simulink model "Case1_Sim"  (R2020b)
settings: Solver=FixedStepAuto  StartTime=0.0  StopTime=0.8  FixedStep=Ts  RelTol=1e-3
values from neighbouring files (symbols this model uses):
  m = 5/100    (= 0.05)    [Case1_SimPara.m]
  Sbase = 1    [Case1_SimPara.m]
  Ts = 1/Fs    (= 0.0001)    [Case1_SimPara.m]
  Vbase = 1    [Case1_SimPara.m]
  w_droop = 10*2*pi    (= 62.8318530718)    [Case1_SimPara.m]
  w_pll = 10*2*pi    (= 62.8318530718)    [Case1_SimPara.m]
  w_tau = 1e3*2*pi    (= 6283.18530718)    [Case1_SimPara.m]
  Wbase = 2*pi*50    (= 314.159265359)    [Case1_SimPara.m]
undefined symbols (not defined in the file or in its folder): DiscIntNeverNeededParam
libraries: SimplexPS x22, powerlib x1
(part 1 of 2)
settings Model: Creator=admin_user  LastModifiedBy=admin_user
settings DataIOCC: ReturnWorkspaceOutputs=off

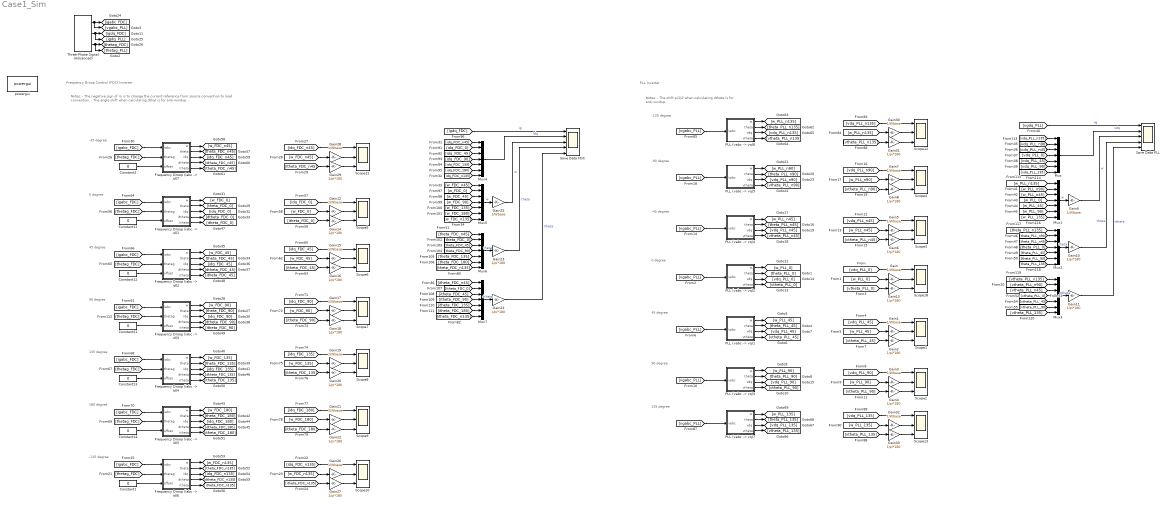
== system Case1_Sim ==
  note: Notes:
      | - The shift pi/2/2 when calculating dtheta is for anti-windup.
  note: Notes:
      | - The negative sign of m is to change the current reference from source convention to load convention.
      | - The angle shift when calculating dthat is for anti-windup.
  note: Frequency Droop Control (FDC) Inverter
  note: 0 degree
  note: PLL Inverter
  note: 90 degree
  note: 0 degree
  note: 45 degree
  note: 135 degree
  note: 180 degree
  note: 45 degree
  note: 90 degree
  note: -45 degree
  note: -90 degree
  note: -135 degree
  note: -45 degree
  note: -135 degree
  note: 135 degree
  Constant{1..2,11..14,21} (7 alike) : Constant  Value=0
  "Frequency Droop (iabc -> id)1" : Subsystem  AncestorBlock=|  mask{Ts=Ts, Sbase=Sbase, Vbase=Vbase, Wbase=Wbase, m=-m, w_tau=w_droop, theta0=0, i0=0, w0=1}
      | SimplexPS/Frequency Droop
      | (iabc -> id)
      mask prompts: Ts "Ts (s), samping period"; Sbase "Sbase (VA), base power"; Vbase "Vbase (V), base voltage"; Wbase "Wbase (rad/s), base angular frequency"; m "m (pu), droop gain"; w_tau "w_tau (rad/s), low-pass filter bandwidth"; theta0 "theta0 (rad), initial angle"; i0 "i0 (pu), current setting point"; w0 "w0 (pu), frequency setting point"
  "Frequency Droop (iabc -> id)2" : Subsystem  AncestorBlock=|  mask{Ts=Ts, Sbase=Sbase, Vbase=Vbase, Wbase=Wbase, m=-m, w_tau=w_droop, theta0=pi/2/2, i0=0, w0=1}
      | SimplexPS/Frequency Droop
      | (iabc -> id)
      mask prompts: Ts "Ts (s), samping period"; Sbase "Sbase (VA), base power"; Vbase "Vbase (V), base voltage"; Wbase "Wbase (rad/s), base angular frequency"; m "m (pu), droop gain"; w_tau "w_tau (rad/s), low-pass filter bandwidth"; theta0 "theta0 (rad), initial angle"; i0 "i0 (pu), current setting point"; w0 "w0 (pu), frequency setting point"
  "Frequency Droop (iabc -> id)3" : Subsystem  AncestorBlock=|  mask{Ts=Ts, Sbase=Sbase, Vbase=Vbase, Wbase=Wbase, m=-m, w_tau=w_droop, theta0=pi/2, i0=0, w0=1}
      | SimplexPS/Frequency Droop
      | (iabc -> id)
      mask prompts: Ts "Ts (s), samping period"; Sbase "Sbase (VA), base power"; Vbase "Vbase (V), base voltage"; Wbase "Wbase (rad/s), base angular frequency"; m "m (pu), droop gain"; w_tau "w_tau (rad/s), low-pass filter bandwidth"; theta0 "theta0 (rad), initial angle"; i0 "i0 (pu), current setting point"; w0 "w0 (pu), frequency setting point"
  "Frequency Droop (iabc -> id)4" : Subsystem  AncestorBlock=|  mask{Ts=Ts, Sbase=Sbase, Vbase=Vbase, Wbase=Wbase, m=-m, w_tau=w_droop, theta0=pi/2/2*3, i0=0, w0=1}
      | SimplexPS/Frequency Droop
      | (iabc -> id)
      mask prompts: Ts "Ts (s), samping period"; Sbase "Sbase (VA), base power"; Vbase "Vbase (V), base voltage"; Wbase "Wbase (rad/s), base angular frequency"; m "m (pu), droop gain"; w_tau "w_tau (rad/s), low-pass filter bandwidth"; theta0 "theta0 (rad), initial angle"; i0 "i0 (pu), current setting point"; w0 "w0 (pu), frequency setting point"
  "Frequency Droop (iabc -> id)5" : Subsystem  AncestorBlock=|  mask{Ts=Ts, Sbase=Sbase, Vbase=Vbase, Wbase=Wbase, m=-m, w_tau=w_droop, theta0=pi, i0=0, w0=1}
      | SimplexPS/Frequency Droop
      | (iabc -> id)
      mask prompts: Ts "Ts (s), samping period"; Sbase "Sbase (VA), base power"; Vbase "Vbase (V), base voltage"; Wbase "Wbase (rad/s), base angular frequency"; m "m (pu), droop gain"; w_tau "w_tau (rad/s), low-pass filter bandwidth"; theta0 "theta0 (rad), initial angle"; i0 "i0 (pu), current setting point"; w0 "w0 (pu), frequency setting point"
  "Frequency Droop (iabc -> id)6" : Subsystem  AncestorBlock=|  mask{Ts=Ts, Sbase=Sbase, Vbase=Vbase, Wbase=Wbase, m=-m, w_tau=w_droop, theta0=-pi/2/2*3, i0=0, w0=1}
      | SimplexPS/Frequency Droop
      | (iabc -> id)
      mask prompts: Ts "Ts (s), samping period"; Sbase "Sbase (VA), base power"; Vbase "Vbase (V), base voltage"; Wbase "Wbase (rad/s), base angular frequency"; m "m (pu), droop gain"; w_tau "w_tau (rad/s), low-pass filter bandwidth"; theta0 "theta0 (rad), initial angle"; i0 "i0 (pu), current setting point"; w0 "w0 (pu), frequency setting point"
  "Frequency Droop (iabc -> id)7" : Subsystem  AncestorBlock=|  mask{Ts=Ts, Sbase=Sbase, Vbase=Vbase, Wbase=Wbase, m=-m, w_tau=w_droop, theta0=-pi/2/2, i0=0, w0=1}
      | SimplexPS/Frequency Droop
      | (iabc -> id)
      mask prompts: Ts "Ts (s), samping period"; Sbase "Sbase (VA), base power"; Vbase "Vbase (V), base voltage"; Wbase "Wbase (rad/s), base angular frequency"; m "m (pu), droop gain"; w_tau "w_tau (rad/s), low-pass filter bandwidth"; theta0 "theta0 (rad), initial angle"; i0 "i0 (pu), current setting point"; w0 "w0 (pu), frequency setting point"
  Gain{,1,3,5,7,9,12,15,17,19,21,25..26,28,30,32} (16 alike) : Gain  Gain=1/Wbase
  Gain{2,4,6,8,10..11,13..14,16,18,20,22..24,27,29,31,33} (18 alike) : Gain  Gain=1/pi*180
  Mux : Mux  Inputs=[2,2,2,2,2,2,2]
  Mux{1..3,5..7} (6 alike) : Mux  Inputs=7
  Mux4 : Mux  Inputs=[2,2,2,2,2,2,2]
  "PLL (vabc -> vq)1" : Subsystem  AncestorBlock=|  mask{Ts=Ts, Vbase=Vbase, Wbase=Wbase, w_pll=w_pll, w_tau=w_tau, theta0=pi/2/2}
      | SimplexPS/PLL
      | (vabc -> vq)
      mask prompts: Ts "Ts (s), sampling period"; Vbase "Vbase (V), base voltage"; Wbase "Wbase (rad/s), base angular frequency"; w_pll "w_pll (rad/s), PLL bandwidth"; w_tau "w_tau (rad/s), low-pass filter bandwidth"; theta0 "theta0 (rad), initial angle"
  "PLL (vabc -> vq)2" : Subsystem  AncestorBlock=|  mask{Ts=Ts, Vbase=Vbase, Wbase=Wbase, w_pll=w_pll, w_tau=w_tau, theta0=0}
      | SimplexPS/PLL
      | (vabc -> vq)
      mask prompts: Ts "Ts (s), sampling period"; Vbase "Vbase (V), base voltage"; Wbase "Wbase (rad/s), base angular frequency"; w_pll "w_pll (rad/s), PLL bandwidth"; w_tau "w_tau (rad/s), low-pass filter bandwidth"; theta0 "theta0 (rad), initial angle"
  "PLL (vabc -> vq)3" : Subsystem  AncestorBlock=|  mask{Ts=Ts, Vbase=Vbase, Wbase=Wbase, w_pll=w_pll, w_tau=w_tau, theta0=pi/2}
      | SimplexPS/PLL
      | (vabc -> vq)
      mask prompts: Ts "Ts (s), sampling period"; Vbase "Vbase (V), base voltage"; Wbase "Wbase (rad/s), base angular frequency"; w_pll "w_pll (rad/s), PLL bandwidth"; w_tau "w_tau (rad/s), low-pass filter bandwidth"; theta0 "theta0 (rad), initial angle"
  "PLL (vabc -> vq)4" : Subsystem  AncestorBlock=|  mask{Ts=Ts, Vbase=Vbase, Wbase=Wbase, w_pll=w_pll, w_tau=w_tau, theta0=-pi/2/2}
      | SimplexPS/PLL
      | (vabc -> vq)
      mask prompts: Ts "Ts (s), sampling period"; Vbase "Vbase (V), base voltage"; Wbase "Wbase (rad/s), base angular frequency"; w_pll "w_pll (rad/s), PLL bandwidth"; w_tau "w_tau (rad/s), low-pass filter bandwidth"; theta0 "theta0 (rad), initial angle"
  "PLL (vabc -> vq)5" : Subsystem  AncestorBlock=|  mask{Ts=Ts, Vbase=Vbase, Wbase=Wbase, w_pll=w_pll, w_tau=w_tau, theta0=-pi/2}
      | SimplexPS/PLL
      | (vabc -> vq)
      mask prompts: Ts "Ts (s), sampling period"; Vbase "Vbase (V), base voltage"; Wbase "Wbase (rad/s), base angular frequency"; w_pll "w_pll (rad/s), PLL bandwidth"; w_tau "w_tau (rad/s), low-pass filter bandwidth"; theta0 "theta0 (rad), initial angle"
  "PLL (vabc -> vq)6" : Subsystem  AncestorBlock=|  mask{Ts=Ts, Vbase=Vbase, Wbase=Wbase, w_pll=w_pll, w_tau=w_tau, theta0=-pi/2/2*3}
      | SimplexPS/PLL
      | (vabc -> vq)
      mask prompts: Ts "Ts (s), sampling period"; Vbase "Vbase (V), base voltage"; Wbase "Wbase (rad/s), base angular frequency"; w_pll "w_pll (rad/s), PLL bandwidth"; w_tau "w_tau (rad/s), low-pass filter bandwidth"; theta0 "theta0 (rad), initial angle"
  "PLL (vabc -> vq)7" : Subsystem  AncestorBlock=|  mask{Ts=Ts, Vbase=Vbase, Wbase=Wbase, w_pll=w_pll, w_tau=w_tau, theta0=pi/2/2*3}
      | SimplexPS/PLL
      | (vabc -> vq)
      mask prompts: Ts "Ts (s), sampling period"; Vbase "Vbase (V), base voltage"; Wbase "Wbase (rad/s), base angular frequency"; w_pll "w_pll (rad/s), PLL bandwidth"; w_tau "w_tau (rad/s), low-pass filter bandwidth"; theta0 "theta0 (rad), initial angle"
  Save Data FDC : Scope  NumInputPorts=5
  Save Data PLL : Scope  NumInputPorts=5
  Scope{1..13,18} (14 alike) : Scope  NumInputPorts=3
  Three-Phase Signal (Advanced) : SimplexPS/Three-Phase Signal (Advanced)  Ts=Ts  ud=1  uq=0  w=Wbase  theta0=0  enable_freq_step=1  ratio_freq_step=0.96  time_freq_step=0.4
      settings: SourceProductName=Simplex Power Systems
  powergui : powerlib/powergui  Priority=1  SimulationMode=Discrete  SampleTime=Ts  frequency=60  Iterations=50  frequencyindice=0  Pbase=100e6  ErrMax=1e-4  UnitsV=kV  UnitsW=MW  buscounter=0  FunctionMessages=off  echomessages=off  EnableUseOfTLC=off  CurrentSourceSwitches=off  DisableSnubberDevices=off  DisableRonSwitches=off  DisableVfSwitches=off  DisplayEquations=off  AutomaticDiscreteSolvers=off  SolverType=Tustin/Backward Euler (TBE)  Interpol=off  ExternalGateDelay=off  methode=off  Ts=100  x0status=blocks  SPID=on  SwTol=0  HookPort=off  NonlinearTolerance=1e-4  nMaxIteration=100  ContinueOnMaxIteration=off  RestoreLinks=warning  ResistiveCurrentMeasurement=off  Frange=[0:2:500]  Ylog=off  Xlog=on  ShowGrid=off  save=off  variable=ZData  structure=0  ZoomFFT=off  StartTime=0.0  cycles=1  DisplayStyle=1  fundamental=60  FreqAxis=off  MaxFrequency=1000  frequencyindicesteady=1  RmsSteady=1  display=off
  wires:
  Three-Phase Signal (Advanced)/2 -> [igdq_PLL], [igdq_FDC]
  "PLL (vabc -> vq)2"/1(w) -> [w_PLL_0]
  "PLL (vabc -> vq)2"/3(vdq) -> [vdq_PLL_0]
  [vdq_PLL_0] -> Scope18/1
  "PLL (vabc -> vq)2"/2(theta) -> [theta_PLL_0]
  Three-Phase Signal (Advanced)/3 -> [thetag_PLL], [thetag_FDC]
  [w_PLL_0] -> Gain/1
  Three-Phase Signal (Advanced)/1 -> [vgabc_PLL], [igabc_FDC]
  [vgabc_PLL] -> "PLL (vabc -> vq)2"/1(vabc)
  [vgdq_PLL] -> Save Data PLL/1  "vg"
  Mux/1 -> Save Data PLL/2  "vdq"
  Mux1/1 -> Gain9/1  "w"
  Gain9/1 -> Save Data PLL/3  "w"
  Mux2/1 -> Gain10/1  "theta"
  Gain10/1 -> Save Data PLL/4  "theta"
  Mux3/1 -> Gain11/1  "dtheta"
  Gain11/1 -> Save Data PLL/5  "vtheta"
  "Frequency Droop (iabc -> id)3"/2(theta) -> [theta_FDC_90]
  [igabc_FDC] -> "Frequency Droop (iabc -> id)3"/1(iabc)
  "Frequency Droop (iabc -> id)3"/3(idq) -> [idq_FDC_90]
  [w_FDC_0] -> Gain12/1
  [idq_FDC_0] -> Scope5/1
  "Frequency Droop (iabc -> id)3"/1(w) -> [w_FDC_90]
  [vtheta_PLL_0] -> Gain13/1
  [itheta_FDC_0] -> Gain14/1
  Mux4/1 -> Save Data FDC/2  "idq"
  [igdq_FDC] -> Save Data FDC/1  "ig"
  Gain24/1 -> Save Data FDC/5  "itheta"
  Mux5/1 -> Gain25/1  "w"
  Gain23/1 -> Save Data FDC/4  "theta"
  Mux7/1 -> Gain24/1  "dtheta"
  Gain25/1 -> Save Data FDC/3  "w"
  Mux6/1 -> Gain23/1  "theta"
  [thetag_FDC] -> "Frequency Droop (iabc -> id)3"/2(thetag)
  Constant21/1 -> "Frequency Droop (iabc -> id)3"/3(offset)
  "Frequency Droop (iabc -> id)3"/4(dtheta) -> [dtheta_FDC_90]
  Gain12/1 -> Scope5/2
  Gain14/1 -> Scope5/3
  Gain16/1 -> Scope6/3
  Gain15/1 -> Scope6/2
  [w_FDC_45] -> Gain15/1
  [idq_FDC_45] -> Scope6/1
  [itheta_FDC_45] -> Gain16/1
  "Frequency Droop (iabc -> id)1"/3(idq) -> [idq_FDC_0]
  "Frequency Droop (iabc -> id)1"/2(theta) -> [theta_FDC_0]
  "Frequency Droop (iabc -> id)1"/1(w) -> [w_FDC_0]
  [thetag_FDC] -> "Frequency Droop (iabc -> id)1"/2(thetag)
  "Frequency Droop (iabc -> id)1"/4(dtheta) -> [dtheta_FDC_0]
  [igabc_FDC] -> "Frequency Droop (iabc -> id)1"/1(iabc)
  Constant11/1 -> "Frequency Droop (iabc -> id)1"/3(offset)
  Constant12/1 -> "Frequency Droop (iabc -> id)2"/3(offset)
  [igabc_FDC] -> "Frequency Droop (iabc -> id)2"/1(iabc)
  "Frequency Droop (iabc -> id)2"/1(w) -> [w_FDC_45]
  "Frequency Droop (iabc -> id)2"/2(theta) -> [theta_FDC_45]
  "Frequency Droop (iabc -> id)2"/3(idq) -> [idq_FDC_45]
  [thetag_FDC] -> "Frequency Droop (iabc -> id)2"/2(thetag)
  "Frequency Droop (iabc -> id)2"/4(dtheta) -> [dtheta_FDC_45]
  Constant13/1 -> "Frequency Droop (iabc -> id)4"/3(offset)
  "Frequency Droop (iabc -> id)4"/4(dtheta) -> [dtheta_FDC_135]
  [thetag_FDC] -> "Frequency Droop (iabc -> id)4"/2(thetag)
  [igabc_FDC] -> "Frequency Droop (iabc -> id)4"/1(iabc)
  "Frequency Droop (iabc -> id)4"/2(theta) -> [theta_FDC_135]
  "Frequency Droop (iabc -> id)4"/1(w) -> [w_FDC_135]
  "Frequency Droop (iabc -> id)4"/3(idq) -> [idq_FDC_135]
  [thetag_FDC] -> "Frequency Droop (iabc -> id)5"/2(thetag)
  "Frequency Droop (iabc -> id)5"/1(w) -> [w_FDC_180]
  [igabc_FDC] -> "Frequency Droop (iabc -> id)5"/1(iabc)
  "Frequency Droop (iabc -> id)5"/2(theta) -> [theta_FDC_180]
  "Frequency Droop (iabc -> id)5"/4(dtheta) -> [dtheta_FDC_180]
  "Frequency Droop (iabc -> id)5"/3(idq) -> [idq_FDC_180]
  Constant14/1 -> "Frequency Droop (iabc -> id)5"/3(offset)
  Gain18/1 -> Scope7/3
  [idq_FDC_90] -> Scope7/1
  [itheta_FDC_90] -> Gain18/1
  Gain17/1 -> Scope7/2
  [w_FDC_90] -> Gain17/1
  [itheta_FDC_135] -> Gain20/1
  Gain19/1 -> Scope8/2
  Gain20/1 -> Scope8/3
  [w_FDC_135] -> Gain19/1
  [idq_FDC_135] -> Scope8/1
  [idq_FDC_180] -> Scope9/1
  [itheta_FDC_180] -> Gain22/1
  Gain22/1 -> Scope9/3
  Gain21/1 -> Scope9/2
  [w_FDC_180] -> Gain21/1
  "Frequency Droop (iabc -> id)1"/5(itheta) -> [itheta_FDC_0]
  "Frequency Droop (iabc -> id)2"/5(itheta) -> [itheta_FDC_45]
  "Frequency Droop (iabc -> id)3"/5(itheta) -> [itheta_FDC_90]
  "Frequency Droop (iabc -> id)4"/5(itheta) -> [itheta_FDC_135]
  "Frequency Droop (iabc -> id)5"/5(itheta) -> [itheta_FDC_180]
  "PLL (vabc -> vq)2"/4(vtheta) -> [vtheta_PLL_0]
  Gain/1 -> Scope18/2
  Gain13/1 -> Scope18/3
  Gain1/1 -> Scope1/2
  Gain2/1 -> Scope1/3
  [w_PLL_45] -> Gain1/1
  "PLL (vabc -> vq)1"/1(w) -> [w_PLL_45]
  "PLL (vabc -> vq)1"/2(theta) -> [theta_PLL_45]
  "PLL (vabc -> vq)1"/3(vdq) -> [vdq_PLL_45]
  [vgabc_PLL] -> "PLL (vabc -> vq)1"/1(vabc)
  [vdq_PLL_45] -> Scope1/1
  "PLL (vabc -> vq)1"/4(vtheta) -> [vtheta_PLL_45]
  [vtheta_PLL_45] -> Gain2/1
  Gain3/1 -> Scope2/2
  Gain4/1 -> Scope2/3
  [w_PLL_90] -> Gain3/1
  "PLL (vabc -> vq)3"/1(w) -> [w_PLL_90]
  "PLL (vabc -> vq)3"/2(theta) -> [theta_PLL_90]
  "PLL (vabc -> vq)3"/3(vdq) -> [vdq_PLL_90]
  [vgabc_PLL] -> "PLL (vabc -> vq)3"/1(vabc)
  [vdq_PLL_90] -> Scope2/1
  "PLL (vabc -> vq)3"/4(vtheta) -> [vtheta_PLL_90]
  [vtheta_PLL_90] -> Gain4/1
  Gain5/1 -> Scope3/2
  Gain6/1 -> Scope3/3
  [w_PLL_n45] -> Gain5/1
  "PLL (vabc -> vq)4"/1(w) -> [w_PLL_n45]
  "PLL (vabc -> vq)4"/2(theta) -> [theta_PLL_n45]
  "PLL (vabc -> vq)4"/3(vdq) -> [vdq_PLL_n45]
  [vgabc_PLL] -> "PLL (vabc -> vq)4"/1(vabc)
  [vdq_PLL_n45] -> Scope3/1
  "PLL (vabc -> vq)4"/4(vtheta) -> [vtheta_PLL_n45]
  [vtheta_PLL_n45] -> Gain6/1
  [w_PLL_n90] -> Gain7/1
  Gain8/1 -> Scope4/3
  "PLL (vabc -> vq)5"/4(vtheta) -> [vtheta_PLL_n90]
  "PLL (vabc -> vq)5"/2(theta) -> [theta_PLL_n90]
  [vdq_PLL_n90] -> Scope4/1
  [vgabc_PLL] -> "PLL (vabc -> vq)5"/1(vabc)
  "PLL (vabc -> vq)5"/1(w) -> [w_PLL_n90]
  [vtheta_PLL_n90] -> Gain8/1
  "PLL (vabc -> vq)5"/3(vdq) -> [vdq_PLL_n90]
  Gain7/1 -> Scope4/2
  "Frequency Droop (iabc -> id)6"/5(itheta) -> [itheta_FDC_n135]
  Gain26/1 -> Scope10/2
  [idq_FDC_n135] -> Scope10/1
  [itheta_FDC_n135] -> Gain27/1
  Constant1/1 -> "Frequency Droop (iabc -> id)6"/3(offset)
  [igabc_FDC] -> "Frequency Droop (iabc -> id)6"/1(iabc)
  "Frequency Droop (iabc -> id)6"/1(w) -> [w_FDC_n135]
  Gain27/1 -> Scope10/3
  "Frequency Droop (iabc -> id)6"/2(theta) -> [theta_FDC_n135]
  [thetag_FDC] -> "Frequency Droop (iabc -> id)6"/2(thetag)
  "Frequency Droop (iabc -> id)6"/4(dtheta) -> [dtheta_FDC_n135]
  [w_FDC_n135] -> Gain26/1
  "Frequency Droop (iabc -> id)6"/3(idq) -> [idq_FDC_n135]
  "Frequency Droop (iabc -> id)7"/1(w) -> [w_FDC_n45]
  [igabc_FDC] -> "Frequency Droop (iabc -> id)7"/1(iabc)
  Constant2/1 -> "Frequency Droop (iabc -> id)7"/3(offset)
  Gain29/1 -> Scope11/3
  "Frequency Droop (iabc -> id)7"/3(idq) -> [idq_FDC_n45]
  [itheta_FDC_n45] -> Gain29/1
  [idq_FDC_n45] -> Scope11/1
  Gain28/1 -> Scope11/2
  "Frequency Droop (iabc -> id)7"/2(theta) -> [theta_FDC_n45]
  "Frequency Droop (iabc -> id)7"/5(itheta) -> [itheta_FDC_n45]
  [w_FDC_n45] -> Gain28/1
  [thetag_FDC] -> "Frequency Droop (iabc -> id)7"/2(thetag)
  "Frequency Droop (iabc -> id)7"/4(dtheta) -> [dtheta_FDC_n45]
  [idq_FDC_n45] -> Mux4/1
  [idq_FDC_0] -> Mux4/2
  [idq_FDC_45] -> Mux4/3
  [idq_FDC_90] -> Mux4/4
  [idq_FDC_135] -> Mux4/5
  [idq_FDC_180] -> Mux4/6
  [idq_FDC_n135] -> Mux4/7
  [w_FDC_n45] -> Mux5/1
  [w_FDC_0] -> Mux5/2
  [w_FDC_45] -> Mux5/3
  [w_FDC_90] -> Mux5/4
  [w_FDC_135] -> Mux5/5
  [w_FDC_180] -> Mux5/6
  [w_FDC_n135] -> Mux5/7
  [theta_FDC_n45] -> Mux6/1
  [theta_FDC_0] -> Mux6/2
  [theta_FDC_45] -> Mux6/3
  [theta_FDC_90] -> Mux6/4
  [theta_FDC_135] -> Mux6/5
  [theta_FDC_180] -> Mux6/6
  [theta_FDC_n135] -> Mux6/7
  [itheta_FDC_n45] -> Mux7/1
  [itheta_FDC_0] -> Mux7/2
  [itheta_FDC_45] -> Mux7/3
  [itheta_FDC_90] -> Mux7/4
  [itheta_FDC_135] -> Mux7/5
  [itheta_FDC_180] -> Mux7/6
  [itheta_FDC_n135] -> Mux7/7
  Gain30/1 -> Scope12/2
  "PLL (vabc -> vq)6"/3(vdq) -> [vdq_PLL_n135]
  "PLL (vabc -> vq)6"/1(w) -> [w_PLL_n135]
  [vgabc_PLL] -> "PLL (vabc -> vq)6"/1(vabc)
  "PLL (vabc -> vq)6"/2(theta) -> [theta_PLL_n135]
  Gain31/1 -> Scope12/3
  [vtheta_PLL_n135] -> Gain31/1
  [vdq_PLL_n135] -> Scope12/1
  "PLL (vabc -> vq)6"/4(vtheta) -> [vtheta_PLL_n135]
  [w_PLL_n135] -> Gain30/1
  "PLL (vabc -> vq)7"/2(theta) -> [theta_PLL_135]
  "PLL (vabc -> vq)7"/4(vtheta) -> [vtheta_PLL_135]
  [vgabc_PLL] -> "PLL (vabc -> vq)7"/1(vabc)
  "PLL (vabc -> vq)7"/3(vdq) -> [vdq_PLL_135]
  [w_PLL_135] -> Gain32/1
  [vtheta_PLL_135] -> Gain33/1
  Gain32/1 -> Scope13/2
  [vdq_PLL_135] -> Scope13/1
  "PLL (vabc -> vq)7"/1(w) -> [w_PLL_135]
  Gain33/1 -> Scope13/3
  [vdq_PLL_n135] -> Mux/1
  [vdq_PLL_n90] -> Mux/2
  [vdq_PLL_n45] -> Mux/3
  [vdq_PLL_0] -> Mux/4
  [vdq_PLL_45] -> Mux/5
  [vdq_PLL_90] -> Mux/6
  [vdq_PLL_135] -> Mux/7
  [w_PLL_n135] -> Mux1/1
  [w_PLL_n90] -> Mux1/2
  [w_PLL_n45] -> Mux1/3
  [w_PLL_0] -> Mux1/4
  [w_PLL_45] -> Mux1/5
  [w_PLL_90] -> Mux1/6
  [w_PLL_135] -> Mux1/7
  [theta_PLL_n135] -> Mux2/1
  [theta_PLL_n90] -> Mux2/2
  [theta_PLL_n45] -> Mux2/3
  [theta_PLL_0] -> Mux2/4
  [theta_PLL_45] -> Mux2/5
  [theta_PLL_90] -> Mux2/6
  [theta_PLL_135] -> Mux2/7
  [vtheta_PLL_n135] -> Mux3/1
  [vtheta_PLL_n90] -> Mux3/2
  [vtheta_PLL_n45] -> Mux3/3
  [vtheta_PLL_0] -> Mux3/4
  [vtheta_PLL_45] -> Mux3/5
  [vtheta_PLL_90] -> Mux3/6
  [vtheta_PLL_135] -> Mux3/7

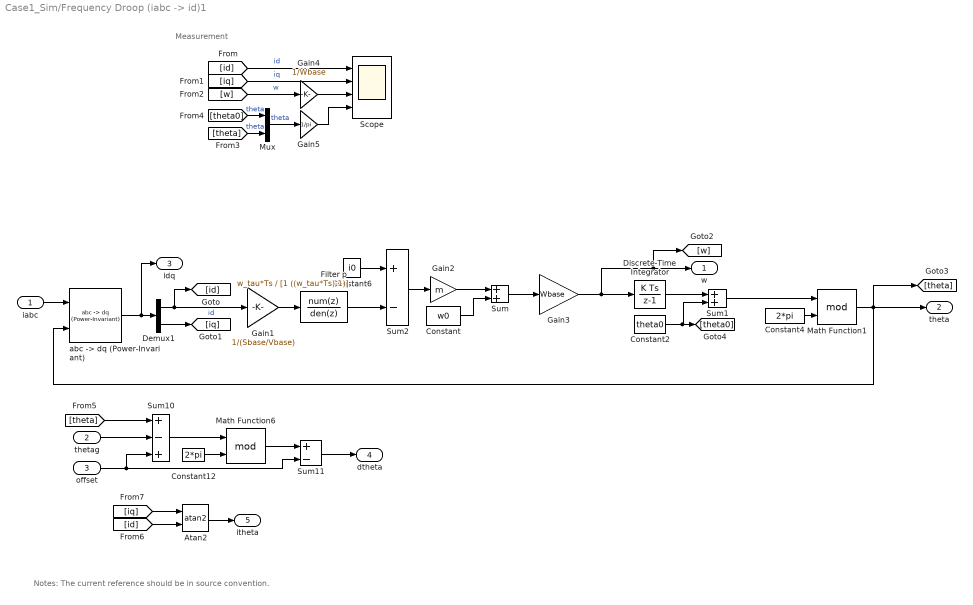
== system Case1_Sim/Frequency Droop (iabc -> id)1 ==
  note: Measurement
  note: Notes: The current reference should be in source convention.
  iabc : Inport
  thetag : Inport  Port=2
  offset : Inport  Port=3
  Atan2 : Trigonometry  Operator=atan2
  Constant : Constant  Value=w0
  Constant12 : Constant  Value=2*pi
  Constant2 : Constant  Value=theta0
  Constant4 : Constant  Value=2*pi
  Constant6 : Constant  Value=i0
  Demux1 : Demux  Outputs=2
  Discrete-Time Integrator : DiscreteIntegrator  SampleTime=Ts  ICPrevOutput=DiscIntNeverNeededParam  ICPrevScaledInput=DiscIntNeverNeededParam
  Filter p : DiscreteTransferFcn  Numerator=w_tau*Ts  Denominator=[1 ((w_tau*Ts)-1)]  SampleTime=Ts
  Gain1 : Gain  Gain=1/(Sbase/Vbase)
  Gain2 : Gain  Gain=m
  Gain3 : Gain  Gain=Wbase
  Gain4 : Gain  Gain=1/Wbase
  Gain5 : Gain  Gain=1/pi
  Math Function1 : Math  Operator=mod  SignedPower=on  SaturateOnIntegerOverflow=on
  Math Function6 : Math  Operator=mod  SignedPower=on  SaturateOnIntegerOverflow=on
  Mux : Mux  Inputs=2
  Scope : Scope  NumInputPorts=4
  Sum : Sum
  Sum1 : Sum
  Sum10 : Sum  Inputs=+-+
  Sum11 : Sum  Inputs=+-
  Sum2 : Sum  Inputs=+-
  "abc -> dq (Power-Invariant)" : SimplexPS/abc -> dq (Power-Invariant)  SystemSampleTime=-1  VariantActivationTime=update diagram  Latency=0  AutoFrameSizeCalculation=off
      settings: SourceProductName=Simplex Power Systems
  w : Outport
  theta : Outport  Port=2
  idq : Outport  Port=3
  dtheta : Outport  Port=4
  itheta : Outport  Port=5
  wires:
  Gain4/1 -> Scope/3
  [w] -> Gain4/1  "w"
  Demux1/2 -> [iq]
  [theta] -> Mux/2  "theta"
  Mux/1 -> Gain5/1  "theta"
  [id] -> Scope/1  "id"
  [theta0] -> Mux/1  "theta"
  [iq] -> Scope/2  "iq"
  Gain5/1 -> Scope/4
  Demux1/1 -> [id], Gain1/1  "id"
  Gain3/1 -> Discrete-Time Integrator/1, w/1, [w]
  Sum/1 -> Gain3/1
  Sum2/1 -> Gain2/1
  Constant6/1 -> Sum2/1
  Gain1/1 -> Filter p/1
  iabc/1 -> "abc -> dq (Power-Invariant)"/1
  Constant4/1 -> Math Function1/2
  "abc -> dq (Power-Invariant)"/1 -> Demux1/1, idq/1
  Constant/1 -> Sum/2
  Filter p/1 -> Sum2/2
  Discrete-Time Integrator/1 -> Sum1/1
  Gain2/1 -> Sum/1
  Math Function1/1 -> theta/1, [theta], "abc -> dq (Power-Invariant)"/2
  Constant2/1 -> [theta0], Sum1/2
  Sum1/1 -> Math Function1/1
  Math Function6/1 -> Sum11/1
  Constant12/1 -> Math Function6/2
  thetag/1 -> Sum10/2
  Sum10/1 -> Math Function6/1
  [theta] -> Sum10/1
  Sum11/1 -> dtheta/1
  offset/1 -> Sum11/2, Sum10/3
  [iq] -> Atan2/1
  [id] -> Atan2/2
  Atan2/1 -> itheta/1

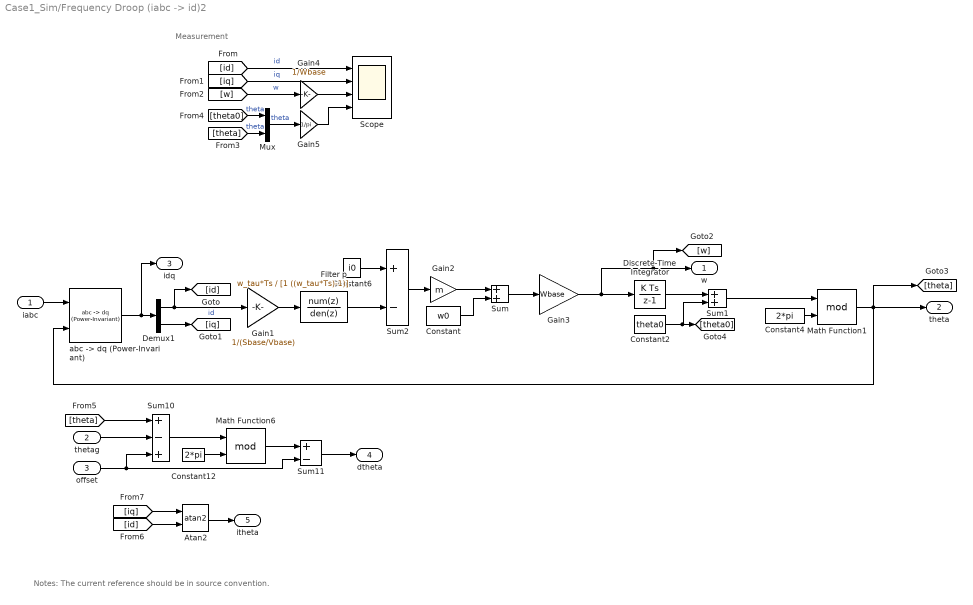
== system Case1_Sim/Frequency Droop (iabc -> id)2 ==
  note: Measurement
  note: Notes: The current reference should be in source convention.
  iabc : Inport
  thetag : Inport  Port=2
  offset : Inport  Port=3
  Atan2 : Trigonometry  Operator=atan2
  Constant : Constant  Value=w0
  Constant12 : Constant  Value=2*pi
  Constant2 : Constant  Value=theta0
  Constant4 : Constant  Value=2*pi
  Constant6 : Constant  Value=i0
  Demux1 : Demux  Outputs=2
  Discrete-Time Integrator : DiscreteIntegrator  SampleTime=Ts  ICPrevOutput=DiscIntNeverNeededParam  ICPrevScaledInput=DiscIntNeverNeededParam
  Filter p : DiscreteTransferFcn  Numerator=w_tau*Ts  Denominator=[1 ((w_tau*Ts)-1)]  SampleTime=Ts
  Gain1 : Gain  Gain=1/(Sbase/Vbase)
  Gain2 : Gain  Gain=m
  Gain3 : Gain  Gain=Wbase
  Gain4 : Gain  Gain=1/Wbase
  Gain5 : Gain  Gain=1/pi
  Math Function1 : Math  Operator=mod  SignedPower=on  SaturateOnIntegerOverflow=on
  Math Function6 : Math  Operator=mod  SignedPower=on  SaturateOnIntegerOverflow=on
  Mux : Mux  Inputs=2
  Scope : Scope  NumInputPorts=4
  Sum : Sum
  Sum1 : Sum
  Sum10 : Sum  Inputs=+-+
  Sum11 : Sum  Inputs=+-
  Sum2 : Sum  Inputs=+-
  "abc -> dq (Power-Invariant)" : SimplexPS/abc -> dq (Power-Invariant)  SystemSampleTime=-1  VariantActivationTime=update diagram  Latency=0  AutoFrameSizeCalculation=off
      settings: SourceProductName=Simplex Power Systems
  w : Outport
  theta : Outport  Port=2
  idq : Outport  Port=3
  dtheta : Outport  Port=4
  itheta : Outport  Port=5
  wires:
  Gain4/1 -> Scope/3
  [w] -> Gain4/1  "w"
  Demux1/2 -> [iq]
  [theta] -> Mux/2  "theta"
  Mux/1 -> Gain5/1  "theta"
  [id] -> Scope/1  "id"
  [theta0] -> Mux/1  "theta"
  [iq] -> Scope/2  "iq"
  Gain5/1 -> Scope/4
  Demux1/1 -> [id], Gain1/1  "id"
  Gain3/1 -> Discrete-Time Integrator/1, w/1, [w]
  Sum/1 -> Gain3/1
  Sum2/1 -> Gain2/1
  Constant6/1 -> Sum2/1
  Gain1/1 -> Filter p/1
  iabc/1 -> "abc -> dq (Power-Invariant)"/1
  Constant4/1 -> Math Function1/2
  "abc -> dq (Power-Invariant)"/1 -> Demux1/1, idq/1
  Constant/1 -> Sum/2
  Filter p/1 -> Sum2/2
  Discrete-Time Integrator/1 -> Sum1/1
  Gain2/1 -> Sum/1
  Math Function1/1 -> theta/1, [theta], "abc -> dq (Power-Invariant)"/2
  Constant2/1 -> [theta0], Sum1/2
  Sum1/1 -> Math Function1/1
  Math Function6/1 -> Sum11/1
  Constant12/1 -> Math Function6/2
  thetag/1 -> Sum10/2
  Sum10/1 -> Math Function6/1
  [theta] -> Sum10/1
  Sum11/1 -> dtheta/1
  offset/1 -> Sum11/2, Sum10/3
  [iq] -> Atan2/1
  [id] -> Atan2/2
  Atan2/1 -> itheta/1

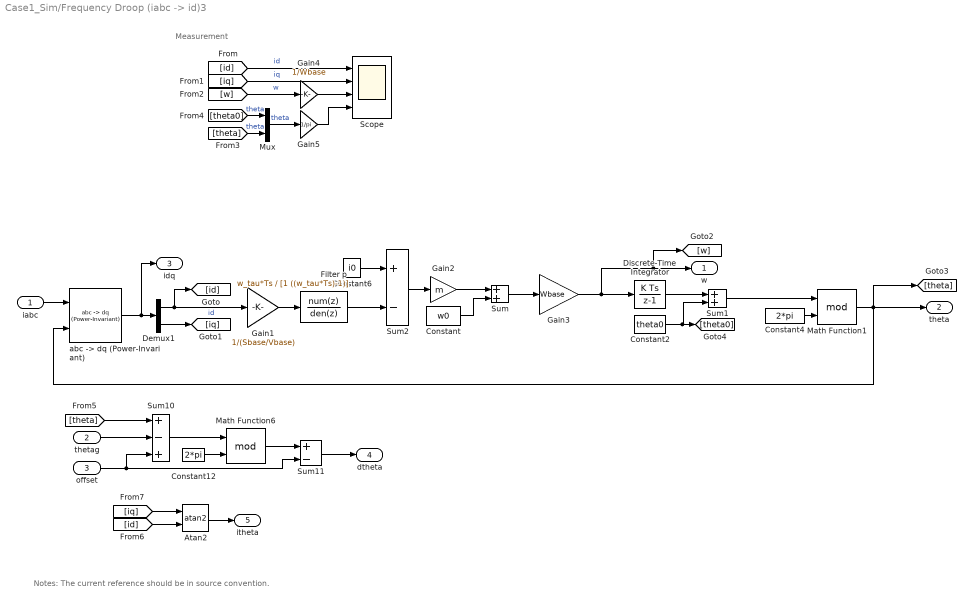
== system Case1_Sim/Frequency Droop (iabc -> id)3 ==
  note: Measurement
  note: Notes: The current reference should be in source convention.
  iabc : Inport
  thetag : Inport  Port=2
  offset : Inport  Port=3
  Atan2 : Trigonometry  Operator=atan2
  Constant : Constant  Value=w0
  Constant12 : Constant  Value=2*pi
  Constant2 : Constant  Value=theta0
  Constant4 : Constant  Value=2*pi
  Constant6 : Constant  Value=i0
  Demux1 : Demux  Outputs=2
  Discrete-Time Integrator : DiscreteIntegrator  SampleTime=Ts  ICPrevOutput=DiscIntNeverNeededParam  ICPrevScaledInput=DiscIntNeverNeededParam
  Filter p : DiscreteTransferFcn  Numerator=w_tau*Ts  Denominator=[1 ((w_tau*Ts)-1)]  SampleTime=Ts
  Gain1 : Gain  Gain=1/(Sbase/Vbase)
  Gain2 : Gain  Gain=m
  Gain3 : Gain  Gain=Wbase
  Gain4 : Gain  Gain=1/Wbase
  Gain5 : Gain  Gain=1/pi
  Math Function1 : Math  Operator=mod  SignedPower=on  SaturateOnIntegerOverflow=on
  Math Function6 : Math  Operator=mod  SignedPower=on  SaturateOnIntegerOverflow=on
  Mux : Mux  Inputs=2
  Scope : Scope  NumInputPorts=4
  Sum : Sum
  Sum1 : Sum
  Sum10 : Sum  Inputs=+-+
  Sum11 : Sum  Inputs=+-
  Sum2 : Sum  Inputs=+-
  "abc -> dq (Power-Invariant)" : SimplexPS/abc -> dq (Power-Invariant)  SystemSampleTime=-1  VariantActivationTime=update diagram  Latency=0  AutoFrameSizeCalculation=off
      settings: SourceProductName=Simplex Power Systems
  w : Outport
  theta : Outport  Port=2
  idq : Outport  Port=3
  dtheta : Outport  Port=4
  itheta : Outport  Port=5
  wires:
  Gain4/1 -> Scope/3
  [w] -> Gain4/1  "w"
  Demux1/2 -> [iq]
  [theta] -> Mux/2  "theta"
  Mux/1 -> Gain5/1  "theta"
  [id] -> Scope/1  "id"
  [theta0] -> Mux/1  "theta"
  [iq] -> Scope/2  "iq"
  Gain5/1 -> Scope/4
  Demux1/1 -> [id], Gain1/1  "id"
  Gain3/1 -> Discrete-Time Integrator/1, w/1, [w]
  Sum/1 -> Gain3/1
  Sum2/1 -> Gain2/1
  Constant6/1 -> Sum2/1
  Gain1/1 -> Filter p/1
  iabc/1 -> "abc -> dq (Power-Invariant)"/1
  Constant4/1 -> Math Function1/2
  "abc -> dq (Power-Invariant)"/1 -> Demux1/1, idq/1
  Constant/1 -> Sum/2
  Filter p/1 -> Sum2/2
  Discrete-Time Integrator/1 -> Sum1/1
  Gain2/1 -> Sum/1
  Math Function1/1 -> theta/1, [theta], "abc -> dq (Power-Invariant)"/2
  Constant2/1 -> [theta0], Sum1/2
  Sum1/1 -> Math Function1/1
  Math Function6/1 -> Sum11/1
  Constant12/1 -> Math Function6/2
  thetag/1 -> Sum10/2
  Sum10/1 -> Math Function6/1
  [theta] -> Sum10/1
  Sum11/1 -> dtheta/1
  offset/1 -> Sum11/2, Sum10/3
  [iq] -> Atan2/1
  [id] -> Atan2/2
  Atan2/1 -> itheta/1

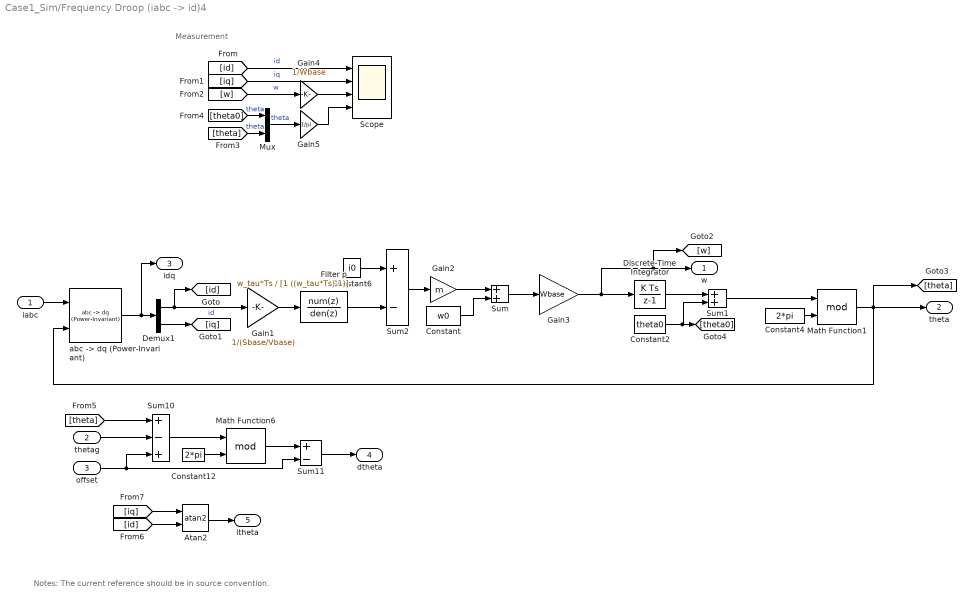
== system Case1_Sim/Frequency Droop (iabc -> id)4 ==
  note: Measurement
  note: Notes: The current reference should be in source convention.
  iabc : Inport
  thetag : Inport  Port=2
  offset : Inport  Port=3
  Atan2 : Trigonometry  Operator=atan2
  Constant : Constant  Value=w0
  Constant12 : Constant  Value=2*pi
  Constant2 : Constant  Value=theta0
  Constant4 : Constant  Value=2*pi
  Constant6 : Constant  Value=i0
  Demux1 : Demux  Outputs=2
  Discrete-Time Integrator : DiscreteIntegrator  SampleTime=Ts  ICPrevOutput=DiscIntNeverNeededParam  ICPrevScaledInput=DiscIntNeverNeededParam
  Filter p : DiscreteTransferFcn  Numerator=w_tau*Ts  Denominator=[1 ((w_tau*Ts)-1)]  SampleTime=Ts
  Gain1 : Gain  Gain=1/(Sbase/Vbase)
  Gain2 : Gain  Gain=m
  Gain3 : Gain  Gain=Wbase
  Gain4 : Gain  Gain=1/Wbase
  Gain5 : Gain  Gain=1/pi
  Math Function1 : Math  Operator=mod  SignedPower=on  SaturateOnIntegerOverflow=on
  Math Function6 : Math  Operator=mod  SignedPower=on  SaturateOnIntegerOverflow=on
  Mux : Mux  Inputs=2
  Scope : Scope  NumInputPorts=4
  Sum : Sum
  Sum1 : Sum
  Sum10 : Sum  Inputs=+-+
  Sum11 : Sum  Inputs=+-
  Sum2 : Sum  Inputs=+-
  "abc -> dq (Power-Invariant)" : SimplexPS/abc -> dq (Power-Invariant)  SystemSampleTime=-1  VariantActivationTime=update diagram  Latency=0  AutoFrameSizeCalculation=off
      settings: SourceProductName=Simplex Power Systems
  w : Outport
  theta : Outport  Port=2
  idq : Outport  Port=3
  dtheta : Outport  Port=4
  itheta : Outport  Port=5
  wires:
  Gain4/1 -> Scope/3
  [w] -> Gain4/1  "w"
  Demux1/2 -> [iq]
  [theta] -> Mux/2  "theta"
  Mux/1 -> Gain5/1  "theta"
  [id] -> Scope/1  "id"
  [theta0] -> Mux/1  "theta"
  [iq] -> Scope/2  "iq"
  Gain5/1 -> Scope/4
  Demux1/1 -> [id], Gain1/1  "id"
  Gain3/1 -> Discrete-Time Integrator/1, w/1, [w]
  Sum/1 -> Gain3/1
  Sum2/1 -> Gain2/1
  Constant6/1 -> Sum2/1
  Gain1/1 -> Filter p/1
  iabc/1 -> "abc -> dq (Power-Invariant)"/1
  Constant4/1 -> Math Function1/2
  "abc -> dq (Power-Invariant)"/1 -> Demux1/1, idq/1
  Constant/1 -> Sum/2
  Filter p/1 -> Sum2/2
  Discrete-Time Integrator/1 -> Sum1/1
  Gain2/1 -> Sum/1
  Math Function1/1 -> theta/1, [theta], "abc -> dq (Power-Invariant)"/2
  Constant2/1 -> [theta0], Sum1/2
  Sum1/1 -> Math Function1/1
  Math Function6/1 -> Sum11/1
  Constant12/1 -> Math Function6/2
  thetag/1 -> Sum10/2
  Sum10/1 -> Math Function6/1
  [theta] -> Sum10/1
  Sum11/1 -> dtheta/1
  offset/1 -> Sum11/2, Sum10/3
  [iq] -> Atan2/1
  [id] -> Atan2/2
  Atan2/1 -> itheta/1

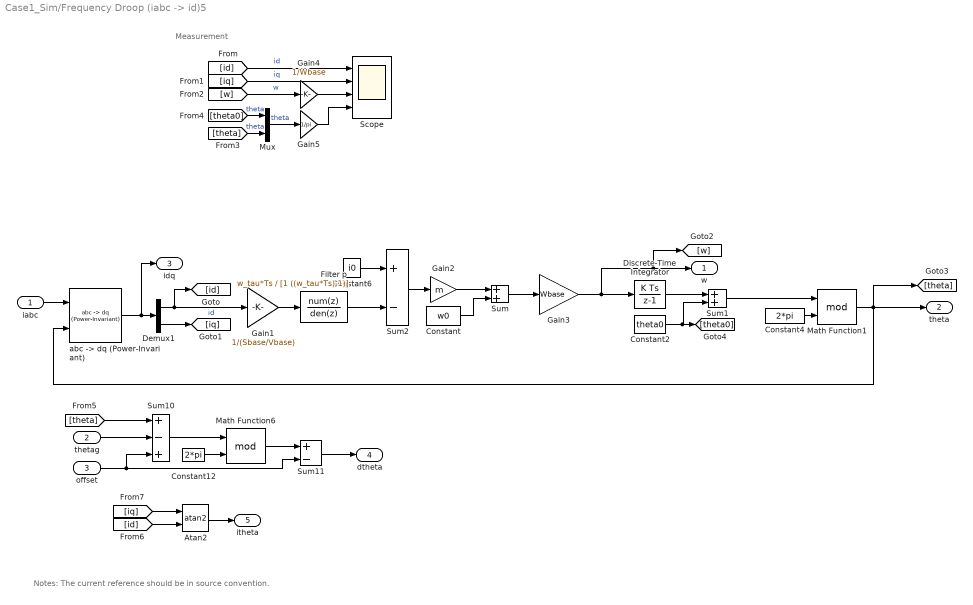
== system Case1_Sim/Frequency Droop (iabc -> id)5 ==
  note: Measurement
  note: Notes: The current reference should be in source convention.
  iabc : Inport
  thetag : Inport  Port=2
  offset : Inport  Port=3
  Atan2 : Trigonometry  Operator=atan2
  Constant : Constant  Value=w0
  Constant12 : Constant  Value=2*pi
  Constant2 : Constant  Value=theta0
  Constant4 : Constant  Value=2*pi
  Constant6 : Constant  Value=i0
  Demux1 : Demux  Outputs=2
  Discrete-Time Integrator : DiscreteIntegrator  SampleTime=Ts  ICPrevOutput=DiscIntNeverNeededParam  ICPrevScaledInput=DiscIntNeverNeededParam
  Filter p : DiscreteTransferFcn  Numerator=w_tau*Ts  Denominator=[1 ((w_tau*Ts)-1)]  SampleTime=Ts
  Gain1 : Gain  Gain=1/(Sbase/Vbase)
  Gain2 : Gain  Gain=m
  Gain3 : Gain  Gain=Wbase
  Gain4 : Gain  Gain=1/Wbase
  Gain5 : Gain  Gain=1/pi
  Math Function1 : Math  Operator=mod  SignedPower=on  SaturateOnIntegerOverflow=on
  Math Function6 : Math  Operator=mod  SignedPower=on  SaturateOnIntegerOverflow=on
  Mux : Mux  Inputs=2
  Scope : Scope  NumInputPorts=4
  Sum : Sum
  Sum1 : Sum
  Sum10 : Sum  Inputs=+-+
  Sum11 : Sum  Inputs=+-
  Sum2 : Sum  Inputs=+-
  "abc -> dq (Power-Invariant)" : SimplexPS/abc -> dq (Power-Invariant)  SystemSampleTime=-1  VariantActivationTime=update diagram  Latency=0  AutoFrameSizeCalculation=off
      settings: SourceProductName=Simplex Power Systems
  w : Outport
  theta : Outport  Port=2
  idq : Outport  Port=3
  dtheta : Outport  Port=4
  itheta : Outport  Port=5
  wires:
  Gain4/1 -> Scope/3
  [w] -> Gain4/1  "w"
  Demux1/2 -> [iq]
  [theta] -> Mux/2  "theta"
  Mux/1 -> Gain5/1  "theta"
  [id] -> Scope/1  "id"
  [theta0] -> Mux/1  "theta"
  [iq] -> Scope/2  "iq"
  Gain5/1 -> Scope/4
  Demux1/1 -> [id], Gain1/1  "id"
  Gain3/1 -> Discrete-Time Integrator/1, w/1, [w]
  Sum/1 -> Gain3/1
  Sum2/1 -> Gain2/1
  Constant6/1 -> Sum2/1
  Gain1/1 -> Filter p/1
  iabc/1 -> "abc -> dq (Power-Invariant)"/1
  Constant4/1 -> Math Function1/2
  "abc -> dq (Power-Invariant)"/1 -> Demux1/1, idq/1
  Constant/1 -> Sum/2
  Filter p/1 -> Sum2/2
  Discrete-Time Integrator/1 -> Sum1/1
  Gain2/1 -> Sum/1
  Math Function1/1 -> theta/1, [theta], "abc -> dq (Power-Invariant)"/2
  Constant2/1 -> [theta0], Sum1/2
  Sum1/1 -> Math Function1/1
  Math Function6/1 -> Sum11/1
  Constant12/1 -> Math Function6/2
  thetag/1 -> Sum10/2
  Sum10/1 -> Math Function6/1
  [theta] -> Sum10/1
  Sum11/1 -> dtheta/1
  offset/1 -> Sum11/2, Sum10/3
  [iq] -> Atan2/1
  [id] -> Atan2/2
  Atan2/1 -> itheta/1

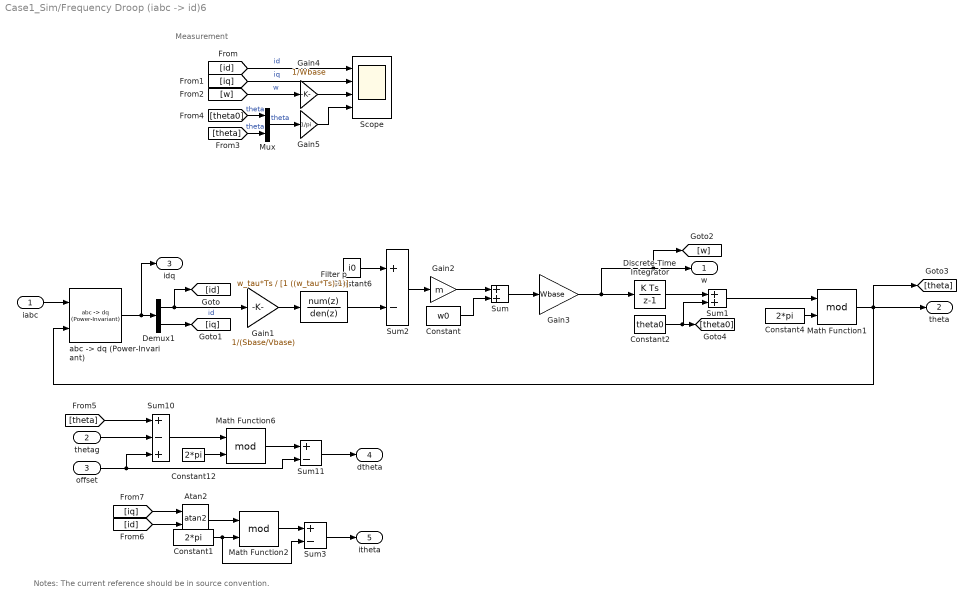
== system Case1_Sim/Frequency Droop (iabc -> id)6 ==
  note: Measurement
  note: Notes: The current reference should be in source convention.
  iabc : Inport
  thetag : Inport  Port=2
  offset : Inport  Port=3
  Atan2 : Trigonometry  Operator=atan2
  Constant : Constant  Value=w0
  Constant1 : Constant  Value=2*pi
  Constant12 : Constant  Value=2*pi
  Constant2 : Constant  Value=theta0
  Constant4 : Constant  Value=2*pi
  Constant6 : Constant  Value=i0
  Demux1 : Demux  Outputs=2
  Discrete-Time Integrator : DiscreteIntegrator  SampleTime=Ts  ICPrevOutput=DiscIntNeverNeededParam  ICPrevScaledInput=DiscIntNeverNeededParam
  Filter p : DiscreteTransferFcn  Numerator=w_tau*Ts  Denominator=[1 ((w_tau*Ts)-1)]  SampleTime=Ts
  Gain1 : Gain  Gain=1/(Sbase/Vbase)
  Gain2 : Gain  Gain=m
  Gain3 : Gain  Gain=Wbase
  Gain4 : Gain  Gain=1/Wbase
  Gain5 : Gain  Gain=1/pi
  Math Function1 : Math  Operator=mod  SignedPower=on  SaturateOnIntegerOverflow=on
  Math Function2 : Math  Operator=mod  SignedPower=on  SaturateOnIntegerOverflow=on
  Math Function6 : Math  Operator=mod  SignedPower=on  SaturateOnIntegerOverflow=on
  Mux : Mux  Inputs=2
  Scope : Scope  NumInputPorts=4
  Sum : Sum
  Sum1 : Sum
  Sum10 : Sum  Inputs=+-+
  Sum11 : Sum  Inputs=+-
  Sum2 : Sum  Inputs=+-
  Sum3 : Sum  Inputs=+-
  "abc -> dq (Power-Invariant)" : SimplexPS/abc -> dq (Power-Invariant)  SystemSampleTime=-1  VariantActivationTime=update diagram  Latency=0  AutoFrameSizeCalculation=off
      settings: SourceProductName=Simplex Power Systems
  w : Outport
  theta : Outport  Port=2
  idq : Outport  Port=3
  dtheta : Outport  Port=4
  itheta : Outport  Port=5
  wires:
  Gain4/1 -> Scope/3
  [w] -> Gain4/1  "w"
  Demux1/2 -> [iq]
  [theta] -> Mux/2  "theta"
  Mux/1 -> Gain5/1  "theta"
  [id] -> Scope/1  "id"
  [theta0] -> Mux/1  "theta"
  [iq] -> Scope/2  "iq"
  Gain5/1 -> Scope/4
  Demux1/1 -> [id], Gain1/1  "id"
  Gain3/1 -> Discrete-Time Integrator/1, w/1, [w]
  Sum/1 -> Gain3/1
  Sum2/1 -> Gain2/1
  Constant6/1 -> Sum2/1
  Gain1/1 -> Filter p/1
  iabc/1 -> "abc -> dq (Power-Invariant)"/1
  Constant4/1 -> Math Function1/2
  "abc -> dq (Power-Invariant)"/1 -> Demux1/1, idq/1
  Constant/1 -> Sum/2
  Filter p/1 -> Sum2/2
  Discrete-Time Integrator/1 -> Sum1/1
  Gain2/1 -> Sum/1
  Math Function1/1 -> theta/1, [theta], "abc -> dq (Power-Invariant)"/2
  Constant2/1 -> [theta0], Sum1/2
  Sum1/1 -> Math Function1/1
  Math Function6/1 -> Sum11/1
  Constant12/1 -> Math Function6/2
  thetag/1 -> Sum10/2
  Sum10/1 -> Math Function6/1
  [theta] -> Sum10/1
  Sum11/1 -> dtheta/1
  offset/1 -> Sum11/2, Sum10/3
  [iq] -> Atan2/1
  [id] -> Atan2/2
  Atan2/1 -> Math Function2/1
  Math Function2/1 -> Sum3/1
  Constant1/1 -> Sum3/2, Math Function2/2
  Sum3/1 -> itheta/1

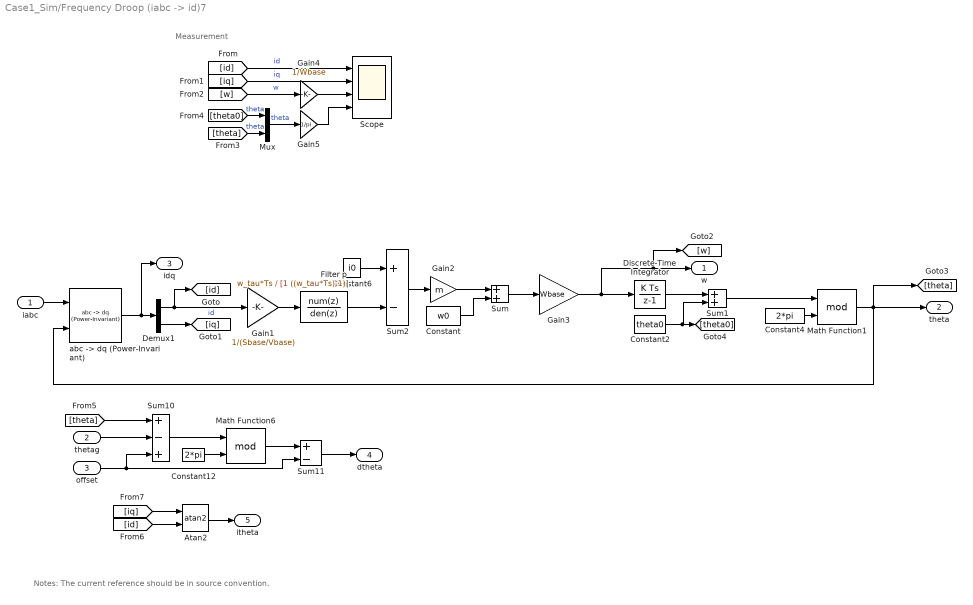
== system Case1_Sim/Frequency Droop (iabc -> id)7 ==
  note: Measurement
  note: Notes: The current reference should be in source convention.
  iabc : Inport
  thetag : Inport  Port=2
  offset : Inport  Port=3
  Atan2 : Trigonometry  Operator=atan2
  Constant : Constant  Value=w0
  Constant12 : Constant  Value=2*pi
  Constant2 : Constant  Value=theta0
  Constant4 : Constant  Value=2*pi
  Constant6 : Constant  Value=i0
  Demux1 : Demux  Outputs=2
  Discrete-Time Integrator : DiscreteIntegrator  SampleTime=Ts  ICPrevOutput=DiscIntNeverNeededParam  ICPrevScaledInput=DiscIntNeverNeededParam
  Filter p : DiscreteTransferFcn  Numerator=w_tau*Ts  Denominator=[1 ((w_tau*Ts)-1)]  SampleTime=Ts
  Gain1 : Gain  Gain=1/(Sbase/Vbase)
  Gain2 : Gain  Gain=m
  Gain3 : Gain  Gain=Wbase
  Gain4 : Gain  Gain=1/Wbase
  Gain5 : Gain  Gain=1/pi
  Math Function1 : Math  Operator=mod  SignedPower=on  SaturateOnIntegerOverflow=on
  Math Function6 : Math  Operator=mod  SignedPower=on  SaturateOnIntegerOverflow=on
  Mux : Mux  Inputs=2
  Scope : Scope  NumInputPorts=4
  Sum : Sum
  Sum1 : Sum
  Sum10 : Sum  Inputs=+-+
  Sum11 : Sum  Inputs=+-
  Sum2 : Sum  Inputs=+-
  "abc -> dq (Power-Invariant)" : SimplexPS/abc -> dq (Power-Invariant)  SystemSampleTime=-1  VariantActivationTime=update diagram  Latency=0  AutoFrameSizeCalculation=off
      settings: SourceProductName=Simplex Power Systems
  w : Outport
  theta : Outport  Port=2
  idq : Outport  Port=3
  dtheta : Outport  Port=4
  itheta : Outport  Port=5
  wires:
  Gain4/1 -> Scope/3
  [w] -> Gain4/1  "w"
  Demux1/2 -> [iq]
  [theta] -> Mux/2  "theta"
  Mux/1 -> Gain5/1  "theta"
  [id] -> Scope/1  "id"
  [theta0] -> Mux/1  "theta"
  [iq] -> Scope/2  "iq"
  Gain5/1 -> Scope/4
  Demux1/1 -> [id], Gain1/1  "id"
  Gain3/1 -> Discrete-Time Integrator/1, w/1, [w]
  Sum/1 -> Gain3/1
  Sum2/1 -> Gain2/1
  Constant6/1 -> Sum2/1
  Gain1/1 -> Filter p/1
  iabc/1 -> "abc -> dq (Power-Invariant)"/1
  Constant4/1 -> Math Function1/2
  "abc -> dq (Power-Invariant)"/1 -> Demux1/1, idq/1
  Constant/1 -> Sum/2
  Filter p/1 -> Sum2/2
  Discrete-Time Integrator/1 -> Sum1/1
  Gain2/1 -> Sum/1
  Math Function1/1 -> theta/1, [theta], "abc -> dq (Power-Invariant)"/2
  Constant2/1 -> [theta0], Sum1/2
  Sum1/1 -> Math Function1/1
  Math Function6/1 -> Sum11/1
  Constant12/1 -> Math Function6/2
  thetag/1 -> Sum10/2
  Sum10/1 -> Math Function6/1
  [theta] -> Sum10/1
  Sum11/1 -> dtheta/1
  offset/1 -> Sum11/2, Sum10/3
  [iq] -> Atan2/1
  [id] -> Atan2/2
  Atan2/1 -> itheta/1

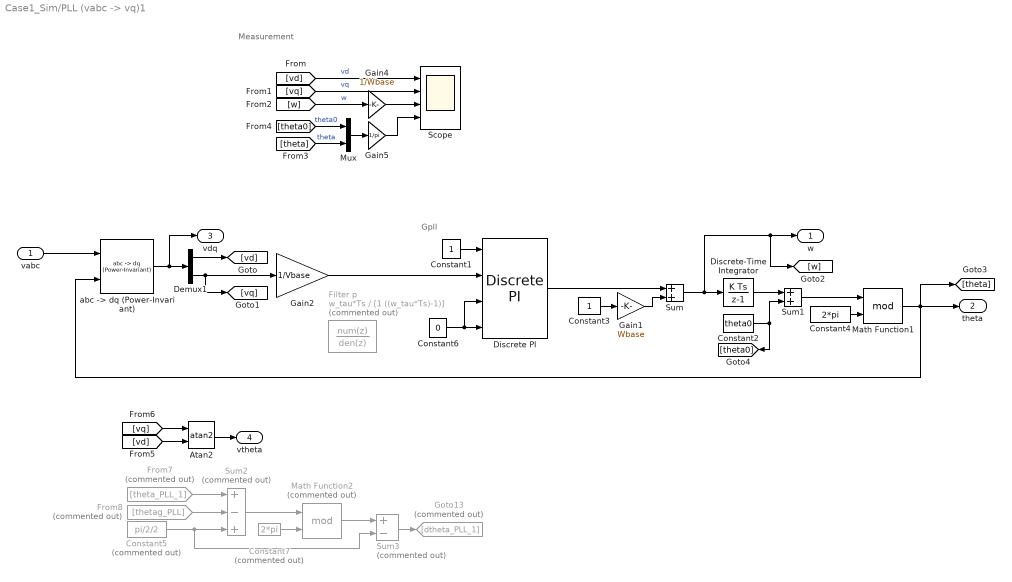
== system Case1_Sim/PLL (vabc -> vq)1 ==
  note: Gpll
  note: Measurement
  vabc : Inport
  Atan2 : Trigonometry  Operator=atan2
  Constant1 : Constant
  Constant2 : Constant  Value=theta0
  Constant3 : Constant
  Constant4 : Constant  Value=2*pi
  Constant5 : Constant  Commented=on  Value=pi/2/2
  Constant6 : Constant  Value=0
  Constant7 : Constant  Commented=on  Value=2*pi
  Demux1 : Demux  Outputs=2
  Discrete PI : SimplexPS/Discrete PI  Kp=w_pll  Ki=w_pll*w_pll/4  xmax=inf  xmin=-inf  Ts=Ts
      settings: SourceProductName=Simplex Power Systems
  Discrete-Time Integrator : DiscreteIntegrator  SampleTime=Ts  ICPrevOutput=DiscIntNeverNeededParam  ICPrevScaledInput=DiscIntNeverNeededParam
  Filter p : DiscreteTransferFcn  Commented=on  Numerator=w_tau*Ts  Denominator=[1 ((w_tau*Ts)-1)]  SampleTime=Ts
  From7 : From  Commented=on  GotoTag=theta_PLL_1
  From8 : From  Commented=on  GotoTag=thetag_PLL
  Gain1 : Gain  Gain=Wbase
  Gain2 : Gain  Gain=1/Vbase
  Gain4 : Gain  Gain=1/Wbase
  Gain5 : Gain  Gain=1/pi
  Goto13 : Goto  Commented=on  GotoTag=dtheta_PLL_1
  Math Function1 : Math  Operator=mod  SignedPower=on  SaturateOnIntegerOverflow=on
  Math Function2 : Math  Commented=on  Operator=mod  SignedPower=on  SaturateOnIntegerOverflow=on
  Mux : Mux  Inputs=2
  Scope : Scope  NumInputPorts=4
  Sum : Sum
  Sum1 : Sum
  Sum2 : Sum  Commented=on  Inputs=+-+
  Sum3 : Sum  Commented=on  Inputs=+-
  "abc -> dq (Power-Invariant)" : SimplexPS/abc -> dq (Power-Invariant)  SystemSampleTime=-1  VariantActivationTime=update diagram  Latency=0  AutoFrameSizeCalculation=off
      settings: SourceProductName=Simplex Power Systems
  w : Outport
  theta : Outport  Port=2
  vdq : Outport  Port=3
  vtheta : Outport  Port=4
  wires:
  Math Function1/1 -> theta/1, [theta], "abc -> dq (Power-Invariant)"/2
  Constant3/1 -> Gain1/1
  Demux1/1 -> [vd]
  [theta] -> Mux/2  "theta"
  Gain5/1 -> Scope/4
  [vd] -> Scope/1  "vd"
  [theta0] -> Mux/1  "theta0"
  [w] -> Gain4/1  "w"
  Gain4/1 -> Scope/3
  Mux/1 -> Gain5/1
  [vq] -> Scope/2  "vq"
  Gain2/1 -> Discrete PI/2
  Constant2/1 -> Sum1/2, [theta0]
  Sum1/1 -> Math Function1/1
  Discrete-Time Integrator/1 -> Sum1/1
  Gain1/1 -> Sum/2
  Sum/1 -> Discrete-Time Integrator/1, w/1, [w]
  Discrete PI/1 -> Sum/1
  Constant1/1 -> Discrete PI/1
  Constant6/1 -> Discrete PI/3, Discrete PI/4
  Demux1/2 -> Gain2/1, [vq]
  Constant4/1 -> Math Function1/2
  "abc -> dq (Power-Invariant)"/1 -> Demux1/1, vdq/1
  vabc/1 -> "abc -> dq (Power-Invariant)"/1
  Atan2/1 -> vtheta/1
  From8/1 -> Sum2/2
  Sum2/1 -> Math Function2/1
  From7/1 -> Sum2/1
  Constant7/1 -> Math Function2/2
  Math Function2/1 -> Sum3/1
  Constant5/1 -> Sum3/2, Sum2/3
  Sum3/1 -> Goto13/1
  [vd] -> Atan2/2
  [vq] -> Atan2/1

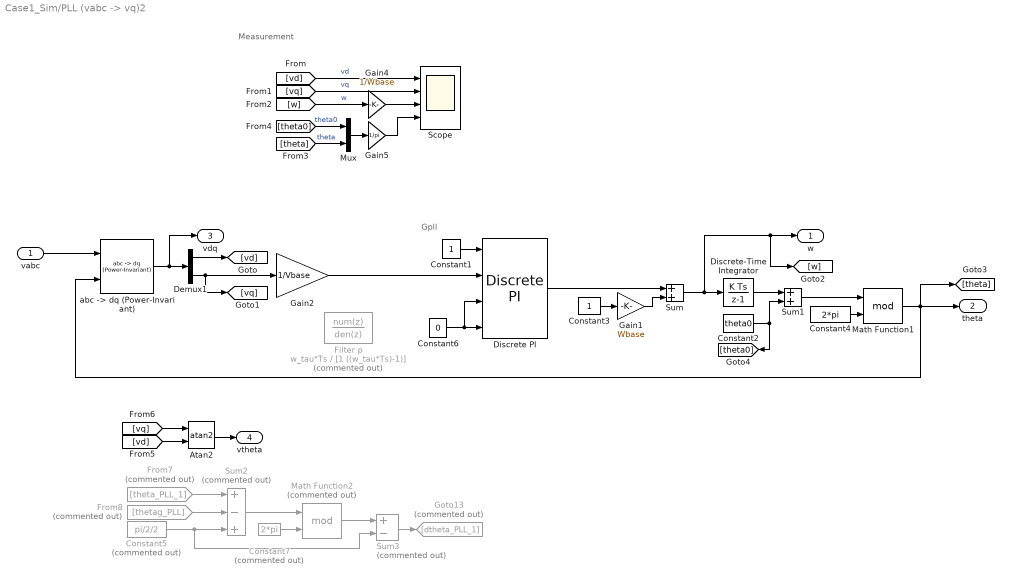
== system Case1_Sim/PLL (vabc -> vq)2 ==
  note: Gpll
  note: Measurement
  vabc : Inport
  Atan2 : Trigonometry  Operator=atan2
  Constant1 : Constant
  Constant2 : Constant  Value=theta0
  Constant3 : Constant
  Constant4 : Constant  Value=2*pi
  Constant5 : Constant  Commented=on  Value=pi/2/2
  Constant6 : Constant  Value=0
  Constant7 : Constant  Commented=on  Value=2*pi
  Demux1 : Demux  Outputs=2
  Discrete PI : SimplexPS/Discrete PI  Kp=w_pll  Ki=w_pll*w_pll/4  xmax=inf  xmin=-inf  Ts=Ts
      settings: SourceProductName=Simplex Power Systems
  Discrete-Time Integrator : DiscreteIntegrator  SampleTime=Ts  ICPrevOutput=DiscIntNeverNeededParam  ICPrevScaledInput=DiscIntNeverNeededParam
  Filter p : DiscreteTransferFcn  Commented=on  Numerator=w_tau*Ts  Denominator=[1 ((w_tau*Ts)-1)]  SampleTime=Ts
  From7 : From  Commented=on  GotoTag=theta_PLL_1
  From8 : From  Commented=on  GotoTag=thetag_PLL
  Gain1 : Gain  Gain=Wbase
  Gain2 : Gain  Gain=1/Vbase
  Gain4 : Gain  Gain=1/Wbase
  Gain5 : Gain  Gain=1/pi
  Goto13 : Goto  Commented=on  GotoTag=dtheta_PLL_1
  Math Function1 : Math  Operator=mod  SignedPower=on  SaturateOnIntegerOverflow=on
  Math Function2 : Math  Commented=on  Operator=mod  SignedPower=on  SaturateOnIntegerOverflow=on
  Mux : Mux  Inputs=2
  Scope : Scope  NumInputPorts=4
  Sum : Sum
  Sum1 : Sum
  Sum2 : Sum  Commented=on  Inputs=+-+
  Sum3 : Sum  Commented=on  Inputs=+-
  "abc -> dq (Power-Invariant)" : SimplexPS/abc -> dq (Power-Invariant)  SystemSampleTime=-1  VariantActivationTime=update diagram  Latency=0  AutoFrameSizeCalculation=off
      settings: SourceProductName=Simplex Power Systems
  w : Outport
  theta : Outport  Port=2
  vdq : Outport  Port=3
  vtheta : Outport  Port=4
  wires:
  Math Function1/1 -> theta/1, [theta], "abc -> dq (Power-Invariant)"/2
  Constant3/1 -> Gain1/1
  Demux1/1 -> [vd]
  [theta] -> Mux/2  "theta"
  Gain5/1 -> Scope/4
  [vd] -> Scope/1  "vd"
  [theta0] -> Mux/1  "theta0"
  [w] -> Gain4/1  "w"
  Gain4/1 -> Scope/3
  Mux/1 -> Gain5/1
  [vq] -> Scope/2  "vq"
  Gain2/1 -> Discrete PI/2
  Constant2/1 -> Sum1/2, [theta0]
  Sum1/1 -> Math Function1/1
  Discrete-Time Integrator/1 -> Sum1/1
  Gain1/1 -> Sum/2
  Sum/1 -> Discrete-Time Integrator/1, w/1, [w]
  Discrete PI/1 -> Sum/1
  Constant1/1 -> Discrete PI/1
  Constant6/1 -> Discrete PI/3, Discrete PI/4
  Demux1/2 -> Gain2/1, [vq]
  Constant4/1 -> Math Function1/2
  "abc -> dq (Power-Invariant)"/1 -> Demux1/1, vdq/1
  vabc/1 -> "abc -> dq (Power-Invariant)"/1
  Atan2/1 -> vtheta/1
  From8/1 -> Sum2/2
  Sum2/1 -> Math Function2/1
  From7/1 -> Sum2/1
  Constant7/1 -> Math Function2/2
  Math Function2/1 -> Sum3/1
  Constant5/1 -> Sum3/2, Sum2/3
  Sum3/1 -> Goto13/1
  [vd] -> Atan2/2
  [vq] -> Atan2/1

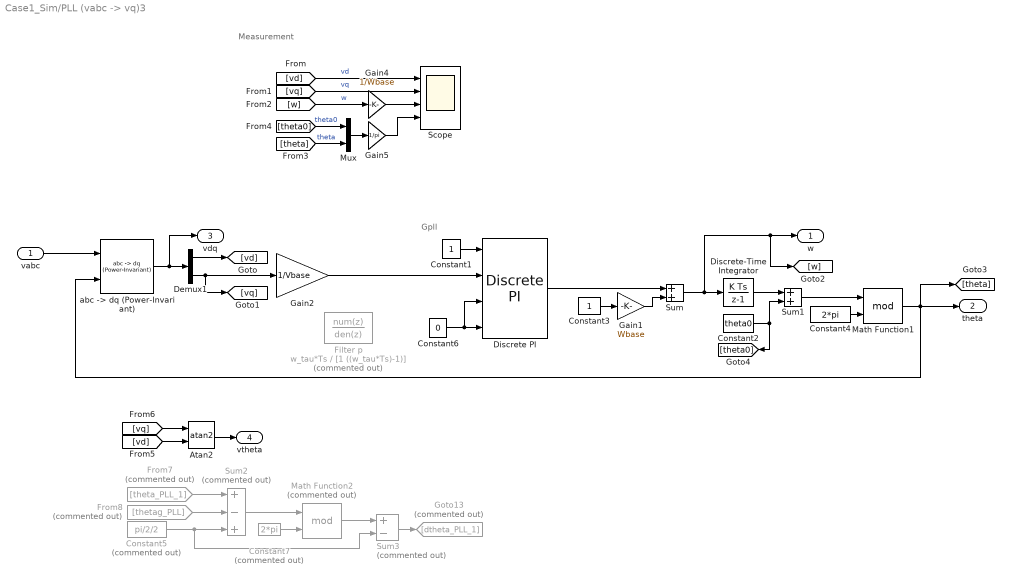
== system Case1_Sim/PLL (vabc -> vq)3 ==
  note: Gpll
  note: Measurement
  vabc : Inport
  Atan2 : Trigonometry  Operator=atan2
  Constant1 : Constant
  Constant2 : Constant  Value=theta0
  Constant3 : Constant
  Constant4 : Constant  Value=2*pi
  Constant5 : Constant  Commented=on  Value=pi/2/2
  Constant6 : Constant  Value=0
  Constant7 : Constant  Commented=on  Value=2*pi
  Demux1 : Demux  Outputs=2
  Discrete PI : SimplexPS/Discrete PI  Kp=w_pll  Ki=w_pll*w_pll/4  xmax=inf  xmin=-inf  Ts=Ts
      settings: SourceProductName=Simplex Power Systems
  Discrete-Time Integrator : DiscreteIntegrator  SampleTime=Ts  ICPrevOutput=DiscIntNeverNeededParam  ICPrevScaledInput=DiscIntNeverNeededParam
  Filter p : DiscreteTransferFcn  Commented=on  Numerator=w_tau*Ts  Denominator=[1 ((w_tau*Ts)-1)]  SampleTime=Ts
  From7 : From  Commented=on  GotoTag=theta_PLL_1
  From8 : From  Commented=on  GotoTag=thetag_PLL
  Gain1 : Gain  Gain=Wbase
  Gain2 : Gain  Gain=1/Vbase
  Gain4 : Gain  Gain=1/Wbase
  Gain5 : Gain  Gain=1/pi
  Goto13 : Goto  Commented=on  GotoTag=dtheta_PLL_1
  Math Function1 : Math  Operator=mod  SignedPower=on  SaturateOnIntegerOverflow=on
  Math Function2 : Math  Commented=on  Operator=mod  SignedPower=on  SaturateOnIntegerOverflow=on
  Mux : Mux  Inputs=2
  Scope : Scope  NumInputPorts=4
  Sum : Sum
  Sum1 : Sum
  Sum2 : Sum  Commented=on  Inputs=+-+
  Sum3 : Sum  Commented=on  Inputs=+-
  "abc -> dq (Power-Invariant)" : SimplexPS/abc -> dq (Power-Invariant)  SystemSampleTime=-1  VariantActivationTime=update diagram  Latency=0  AutoFrameSizeCalculation=off
      settings: SourceProductName=Simplex Power Systems
  w : Outport
  theta : Outport  Port=2
  vdq : Outport  Port=3
  vtheta : Outport  Port=4
  wires:
  Math Function1/1 -> theta/1, [theta], "abc -> dq (Power-Invariant)"/2
  Constant3/1 -> Gain1/1
  Demux1/1 -> [vd]
  [theta] -> Mux/2  "theta"
  Gain5/1 -> Scope/4
  [vd] -> Scope/1  "vd"
  [theta0] -> Mux/1  "theta0"
  [w] -> Gain4/1  "w"
  Gain4/1 -> Scope/3
  Mux/1 -> Gain5/1
  [vq] -> Scope/2  "vq"
  Gain2/1 -> Discrete PI/2
  Constant2/1 -> Sum1/2, [theta0]
  Sum1/1 -> Math Function1/1
  Discrete-Time Integrator/1 -> Sum1/1
  Gain1/1 -> Sum/2
  Sum/1 -> Discrete-Time Integrator/1, w/1, [w]
  Discrete PI/1 -> Sum/1
  Constant1/1 -> Discrete PI/1
  Constant6/1 -> Discrete PI/3, Discrete PI/4
  Demux1/2 -> Gain2/1, [vq]
  Constant4/1 -> Math Function1/2
  "abc -> dq (Power-Invariant)"/1 -> Demux1/1, vdq/1
  vabc/1 -> "abc -> dq (Power-Invariant)"/1
  Atan2/1 -> vtheta/1
  From8/1 -> Sum2/2
  Sum2/1 -> Math Function2/1
  From7/1 -> Sum2/1
  Constant7/1 -> Math Function2/2
  Math Function2/1 -> Sum3/1
  Constant5/1 -> Sum3/2, Sum2/3
  Sum3/1 -> Goto13/1
  [vd] -> Atan2/2
  [vq] -> Atan2/1

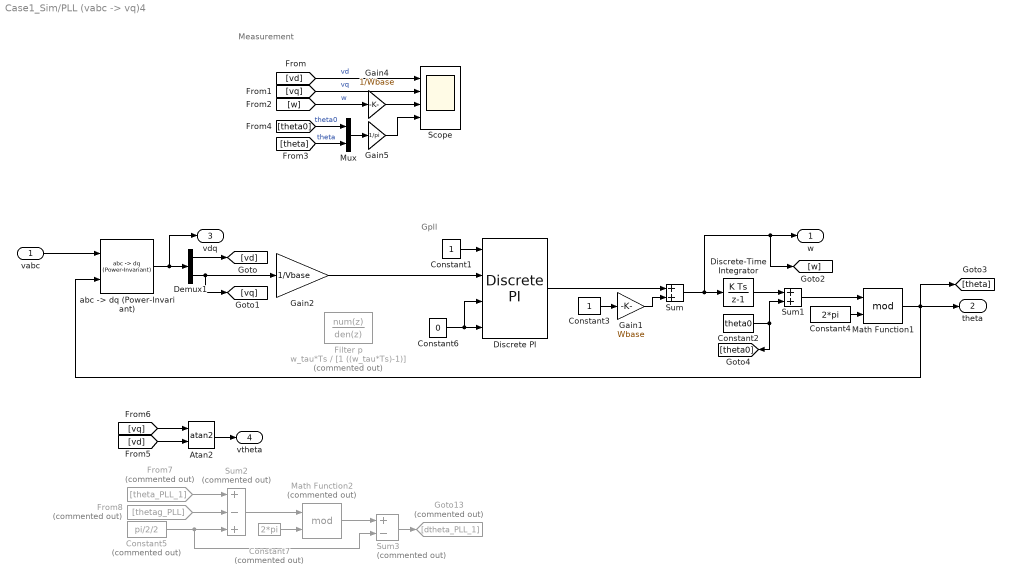
== system Case1_Sim/PLL (vabc -> vq)4 ==
  note: Gpll
  note: Measurement
  vabc : Inport
  Atan2 : Trigonometry  Operator=atan2
  Constant1 : Constant
  Constant2 : Constant  Value=theta0
  Constant3 : Constant
  Constant4 : Constant  Value=2*pi
  Constant5 : Constant  Commented=on  Value=pi/2/2
  Constant6 : Constant  Value=0
  Constant7 : Constant  Commented=on  Value=2*pi
  Demux1 : Demux  Outputs=2
  Discrete PI : SimplexPS/Discrete PI  Kp=w_pll  Ki=w_pll*w_pll/4  xmax=inf  xmin=-inf  Ts=Ts
      settings: SourceProductName=Simplex Power Systems
  Discrete-Time Integrator : DiscreteIntegrator  SampleTime=Ts  ICPrevOutput=DiscIntNeverNeededParam  ICPrevScaledInput=DiscIntNeverNeededParam
  Filter p : DiscreteTransferFcn  Commented=on  Numerator=w_tau*Ts  Denominator=[1 ((w_tau*Ts)-1)]  SampleTime=Ts
  From7 : From  Commented=on  GotoTag=theta_PLL_1
  From8 : From  Commented=on  GotoTag=thetag_PLL
  Gain1 : Gain  Gain=Wbase
  Gain2 : Gain  Gain=1/Vbase
  Gain4 : Gain  Gain=1/Wbase
  Gain5 : Gain  Gain=1/pi
  Goto13 : Goto  Commented=on  GotoTag=dtheta_PLL_1
  Math Function1 : Math  Operator=mod  SignedPower=on  SaturateOnIntegerOverflow=on
  Math Function2 : Math  Commented=on  Operator=mod  SignedPower=on  SaturateOnIntegerOverflow=on
  Mux : Mux  Inputs=2
  Scope : Scope  NumInputPorts=4
  Sum : Sum
  Sum1 : Sum
  Sum2 : Sum  Commented=on  Inputs=+-+
  Sum3 : Sum  Commented=on  Inputs=+-
  "abc -> dq (Power-Invariant)" : SimplexPS/abc -> dq (Power-Invariant)  SystemSampleTime=-1  VariantActivationTime=update diagram  Latency=0  AutoFrameSizeCalculation=off
      settings: SourceProductName=Simplex Power Systems
  w : Outport
  theta : Outport  Port=2
  vdq : Outport  Port=3
  vtheta : Outport  Port=4
  wires:
  Math Function1/1 -> theta/1, [theta], "abc -> dq (Power-Invariant)"/2
  Constant3/1 -> Gain1/1
  Demux1/1 -> [vd]
  [theta] -> Mux/2  "theta"
  Gain5/1 -> Scope/4
  [vd] -> Scope/1  "vd"
  [theta0] -> Mux/1  "theta0"
  [w] -> Gain4/1  "w"
  Gain4/1 -> Scope/3
  Mux/1 -> Gain5/1
  [vq] -> Scope/2  "vq"
  Gain2/1 -> Discrete PI/2
  Constant2/1 -> Sum1/2, [theta0]
  Sum1/1 -> Math Function1/1
  Discrete-Time Integrator/1 -> Sum1/1
  Gain1/1 -> Sum/2
  Sum/1 -> Discrete-Time Integrator/1, w/1, [w]
  Discrete PI/1 -> Sum/1
  Constant1/1 -> Discrete PI/1
  Constant6/1 -> Discrete PI/3, Discrete PI/4
  Demux1/2 -> Gain2/1, [vq]
  Constant4/1 -> Math Function1/2
  "abc -> dq (Power-Invariant)"/1 -> Demux1/1, vdq/1
  vabc/1 -> "abc -> dq (Power-Invariant)"/1
  Atan2/1 -> vtheta/1
  From8/1 -> Sum2/2
  Sum2/1 -> Math Function2/1
  From7/1 -> Sum2/1
  Constant7/1 -> Math Function2/2
  Math Function2/1 -> Sum3/1
  Constant5/1 -> Sum3/2, Sum2/3
  Sum3/1 -> Goto13/1
  [vq] -> Atan2/1
  [vd] -> Atan2/2
